simulink model "Edge_detector"  (Simulink 6.3)
settings: Solver=FixedStepDiscrete  SolverMode=SingleTasking  StartTime=0.0  StopTime=307201.0  RelTol=1e-3
InitFcn:
  | ed_in_script
  | %% DSPBuilder Start
  | alt_dspbuilder_update_model(bdroot)
  | %% DSPBuilder End
StopFcn:
  | ed_out_script
libraries: allblocks_alteradspbuilder2 x46
settings Model: LastModifiedBy=LKONG
settings DataIOCC: SignalLoggingName=sigsOut
settings OptimizationCC: InlineInvariantSignals=on
settings DebuggingCC: SolverPrmCheckMsg=none
settings HardwareCC: TargetUnknown=on

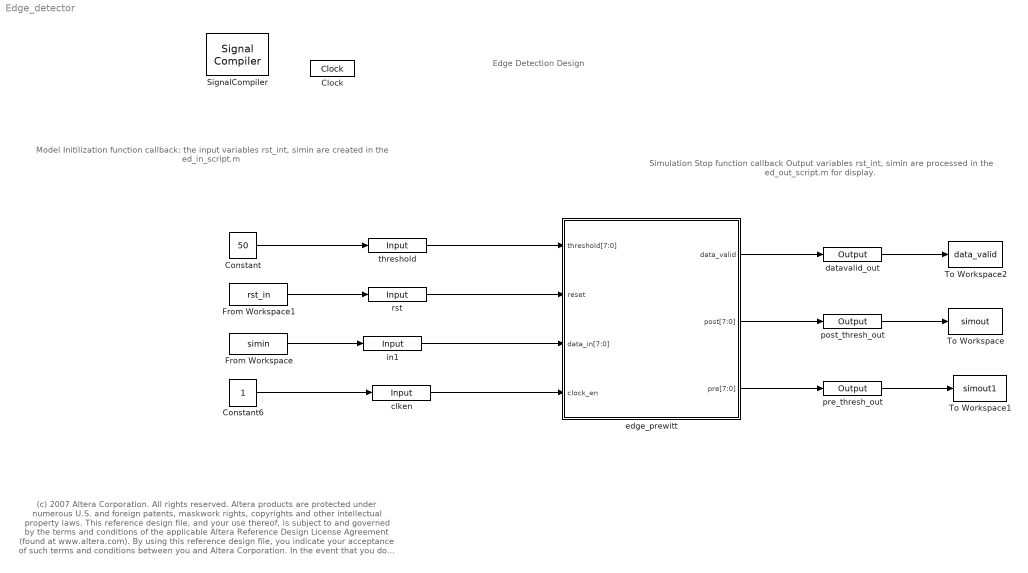
== system Edge_detector ==
  note: Edge Detection Design
  note: (c) 2007 Altera Corporation. All rights reserved.  Altera products are protected under numerous U.S. and foreign patents, maskwork rights, copyrights and other intellectual property laws.
      | This reference design file, and your use thereof, is subject to and governed by the terms and conditions of the applicable Altera Reference Design License Agreement (found at www.altera.com).
      | By using this reference design file, you indicate your acceptance of such terms and conditions between you and Altera Corporation.
      | In the event that you do not agree with such terms and conditions, you may not use the reference design file and please promptly destroy any copies you have made.
      | This reference design file being provided on an "as-is" basis and as an accommodation and therefore all warranties, representations or guarantees of any kind (whether express, implied or statutory)
      | including, without limitation, warranties of merchantability, non-infringement, or fitness for a particular purpose, are specifically disclaimed.
      | By making this reference design file available, Altera expressly does not recommend, suggest or require that this reference design file be used in combination with any other product not provided by Altera
  note: Model Initilization function callback:
      | the input  variables rst_int, simin
      | are created in the ed_in_script.m
  note: Simulation Stop function callback
      | Output  variables rst_int, simin
      | are processed in the ed_out_script.m
      | for display.
  Clock : allblocks_alteradspbuilder2/Clock  ClockPeriod=100  ClockPeriodUnit=ns  SampleTime=1  SimulationStartCycle=5  PhaseOffset=0  Reset=aclr  ResetType=Active Low  Export=off
  Constant : Constant  Value=50
  Constant6 : Constant
  From Workspace : FromWorkspace  VariableName=simin  SampleTime=1
  From Workspace1 : FromWorkspace  VariableName=rst_in  SampleTime=1
  SignalCompiler : allblocks_alteradspbuilder2/Signal Compiler  DeviceFamily=Stratix III  DeviceName=AUTO  EnableSignalTap=off  SignalTapDepth=1024  UseBoardBlock=off  StpUseDefaultClock=on  StpClock=clock
  To Workspace : ToWorkspace  VariableName=simout  SaveFormat=Array
  To Workspace1 : ToWorkspace  VariableName=simout1  SaveFormat=Array
  To Workspace2 : ToWorkspace  VariableName=data_valid  SaveFormat=Array
  clken : allblocks_alteradspbuilder2/Input  iofile=d:\wsTrunk\workspace\Documentation\DesignExamples\Demos\Video\EdgeDetection\tb_Edge_detector\Edge_detector_clken.salt  BusType=Single Bit  bwl=1  bwr=0  SpecifyClock=off  PORTTYPE=Input
  datavalid_out : allblocks_alteradspbuilder2/Output  iofile=d:\wsTrunk\workspace\Documentation\DesignExamples\Demos\Video\EdgeDetection\tb_Edge_detector\Edge_detector_datavalid_out.capture  BusType=Single Bit  bwl=1  bwr=0  PORTTYPE=Output
  edge_prewitt : Subsystem
      mask Type: SubSystem AlteraBlockSet
  in1 : allblocks_alteradspbuilder2/Input  iofile=d:\wsTrunk\workspace\Documentation\DesignExamples\Demos\Video\EdgeDetection\tb_Edge_detector\Edge_detector_in1.salt  BusType=Unsigned Integer  bwl=8  bwr=0  SpecifyClock=off  PORTTYPE=Input
  post_thresh_out : allblocks_alteradspbuilder2/Output  iofile=d:\wsTrunk\workspace\Documentation\DesignExamples\Demos\Video\EdgeDetection\tb_Edge_detector\Edge_detector_post_thresh_out.capture  BusType=Unsigned Integer  bwl=8  bwr=0  PORTTYPE=Output
  pre_thresh_out : allblocks_alteradspbuilder2/Output  iofile=d:\wsTrunk\workspace\Documentation\DesignExamples\Demos\Video\EdgeDetection\tb_Edge_detector\Edge_detector_pre_thresh_out.capture  BusType=Unsigned Integer  bwl=8  bwr=0  PORTTYPE=Output
  rst : allblocks_alteradspbuilder2/Input  iofile=d:\wsTrunk\workspace\Documentation\DesignExamples\Demos\Video\EdgeDetection\tb_Edge_detector\Edge_detector_rst.salt  BusType=Single Bit  bwl=1  bwr=0  SpecifyClock=off  PORTTYPE=Input
  threshold : allblocks_alteradspbuilder2/Input  iofile=d:\wsTrunk\workspace\Documentation\DesignExamples\Demos\Video\EdgeDetection\tb_Edge_detector\Edge_detector_threshold.salt  BusType=Unsigned Integer  bwl=8  bwr=0  SpecifyClock=off  PORTTYPE=Input
  wires:
  Constant6/1 -> clken/1
  Constant/1 -> threshold/1
  From Workspace1/1 -> rst/1
  clken/1 -> edge_prewitt/4(clock_en)
  From Workspace/1 -> in1/1
  in1/1 -> edge_prewitt/3(data_in[7:0])
  rst/1 -> edge_prewitt/2(reset)
  threshold/1 -> edge_prewitt/1(threshold[7:0])
  datavalid_out/1 -> To Workspace2/1
  edge_prewitt/2(post[7:0]) -> post_thresh_out/1
  edge_prewitt/1(data_valid) -> datavalid_out/1
  pre_thresh_out/1 -> To Workspace1/1
  post_thresh_out/1 -> To Workspace/1
  edge_prewitt/3(pre[7:0]) -> pre_thresh_out/1

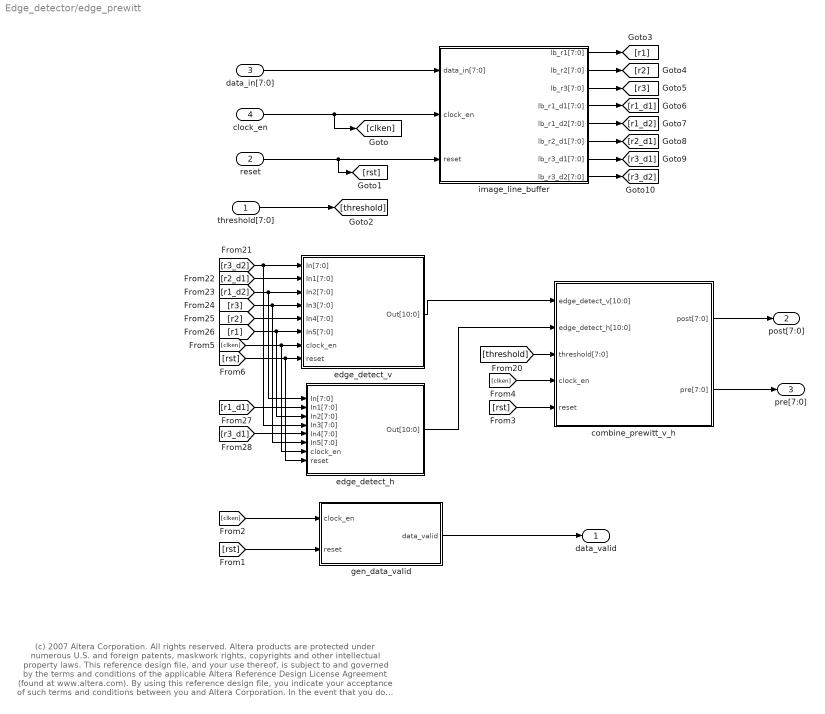
== system Edge_detector/edge_prewitt ==
  note: (c) 2007 Altera Corporation. All rights reserved.  Altera products are protected under numerous U.S. and foreign patents, maskwork rights, copyrights and other intellectual property laws.
      | This reference design file, and your use thereof, is subject to and governed by the terms and conditions of the applicable Altera Reference Design License Agreement (found at www.altera.com).
      | By using this reference design file, you indicate your acceptance of such terms and conditions between you and Altera Corporation.
      | In the event that you do not agree with such terms and conditions, you may not use the reference design file and please promptly destroy any copies you have made.
      | This reference design file being provided on an "as-is" basis and as an accommodation and therefore all warranties, representations or guarantees of any kind (whether express, implied or statutory)
      | including, without limitation, warranties of merchantability, non-infringement, or fitness for a particular purpose, are specifically disclaimed.
      | By making this reference design file available, Altera expressly does not recommend, suggest or require that this reference design file be used in combination with any other product not provided by Altera
  threshold[7:0] : Inport
  reset : Inport  Port=2
  data_in[7:0] : Inport  Port=3
  clock_en : Inport  Port=4
  combine_prewitt_v_h : Subsystem
      mask Type: SubSystem AlteraBlockSet
  edge_detect_h : Subsystem  AncestorBlock=ALTELINK/AltLab/HDL SubSystem
      mask Type: SubSystem AlteraBlockSet
  edge_detect_v : Subsystem  AncestorBlock=ALTELINK/AltLab/HDL SubSystem
      mask Type: SubSystem AlteraBlockSet
  gen_data_valid : Subsystem
      mask Type: SubSystem AlteraBlockSet
  image_line_buffer : Subsystem
      mask Type: SubSystem AlteraBlockSet
  data_valid : Outport
  post[7:0] : Outport  Port=2
  pre[7:0] : Outport  Port=3
  wires:
  threshold[7:0]/1 -> [threshold]
  edge_detect_v/1(Out[10:0]) -> combine_prewitt_v_h/1(edge_detect_v[10:0])
  edge_detect_h/1(Out[10:0]) -> combine_prewitt_v_h/2(edge_detect_h[10:0])
  [r3_d2] -> edge_detect_v/1(In[7:0]), edge_detect_h/4(In3[7:0])
  [r2_d1] -> edge_detect_v/2(In1[7:0])
  [r1_d2] -> edge_detect_v/3(In2[7:0]), edge_detect_h/1(In[7:0])
  [r3] -> edge_detect_v/4(In3[7:0]), edge_detect_h/6(In5[7:0])
  [r2] -> edge_detect_v/5(In4[7:0])
  [r1] -> edge_detect_v/6(In5[7:0]), edge_detect_h/3(In2[7:0])
  [r1_d1] -> edge_detect_h/2(In1[7:0])
  [r3_d1] -> edge_detect_h/5(In4[7:0])
  gen_data_valid/1(data_valid) -> data_valid/1
  image_line_buffer/1(lb_r1[7:0]) -> [r1]
  image_line_buffer/2(lb_r2[7:0]) -> [r2]
  image_line_buffer/3(lb_r3[7:0]) -> [r3]
  image_line_buffer/4(lb_r1_d1[7:0]) -> [r1_d1]
  image_line_buffer/5(lb_r1_d2[7:0]) -> [r1_d2]
  image_line_buffer/6(lb_r2_d1[7:0]) -> [r2_d1]
  image_line_buffer/7(lb_r3_d1[7:0]) -> [r3_d1]
  image_line_buffer/8(lb_r3_d2[7:0]) -> [r3_d2]
  [clken] -> gen_data_valid/1(clock_en)
  [rst] -> gen_data_valid/2(reset)
  [threshold] -> combine_prewitt_v_h/3(threshold[7:0])
  [clken] -> combine_prewitt_v_h/4(clock_en)
  [rst] -> combine_prewitt_v_h/5(reset)
  combine_prewitt_v_h/2(pre[7:0]) -> pre[7:0]/1
  combine_prewitt_v_h/1(post[7:0]) -> post[7:0]/1
  reset/1 -> image_line_buffer/3(reset), [rst]
  data_in[7:0]/1 -> image_line_buffer/1(data_in[7:0])
  clock_en/1 -> image_line_buffer/2(clock_en), [clken]
  [clken] -> edge_detect_v/7(clock_en), edge_detect_h/7(clock_en)
  [rst] -> edge_detect_v/8(reset), edge_detect_h/8(reset)

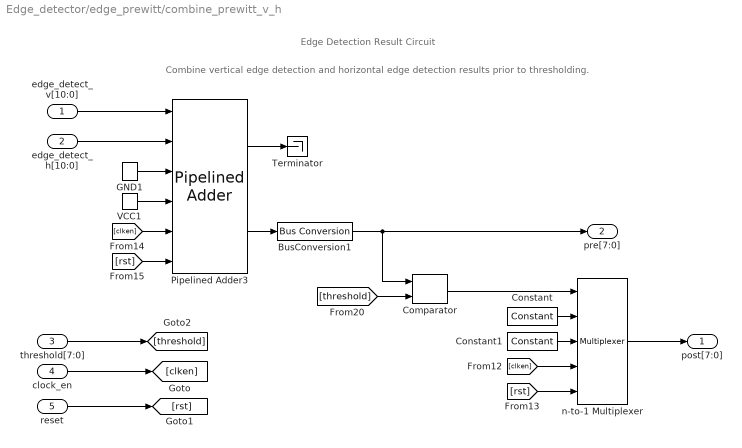
== system Edge_detector/edge_prewitt/combine_prewitt_v_h ==
  note: Combine vertical edge detection and horizontal edge detection results prior to thresholding.
  note: Edge Detection Result Circuit
  edge_detect_v[10:0] : Inport
  edge_detect_h[10:0] : Inport  Port=2
  threshold[7:0] : Inport  Port=3
  clock_en : Inport  Port=4
  reset : Inport  Port=5
  BusConversion1 : allblocks_alteradspbuilder2/Bus Conversion  BusType=Unsigned Integer  ibwl=11  ibwr=0  bwl=8  bwr=0  bitToConnectToOutputLSB=0  round=off  saturate=on
  Comparator : allblocks_alteradspbuilder2/Comparator  direction=a < b
  Constant : allblocks_alteradspbuilder2/Constant  mask_cst=255  BusType=Unsigned Integer  bwl=8  bwr=0  SpecifyClock=off
  Constant1 : allblocks_alteradspbuilder2/Constant  mask_cst=0  BusType=Unsigned Integer  bwl=8  bwr=0  SpecifyClock=off
  GND1 : allblocks_alteradspbuilder2/GND  SpecifyClock=off
  Pipelined Adder3 : allblocks_alteradspbuilder2/Pipelined Adder  BusType=Unsigned Integer  bwl=11  bwr=0  pipeline=1  AddSubDirection=ADD  use_cin=on  use_ovl=on  use_addsub=on  use_ena=on  use_aclr=on
  Terminator : Terminator
  VCC1 : allblocks_alteradspbuilder2/VCC  SpecifyClock=off
  n-to-1 Multiplexer : allblocks_alteradspbuilder2/Multiplexer  numInputs=2  pipeline=1  oneHot=off  use_ena=on  use_aclr=on
  post[7:0] : Outport
  pre[7:0] : Outport  Port=2
  wires:
  Comparator/1 -> n-to-1 Multiplexer/1
  Constant/1 -> n-to-1 Multiplexer/2
  Constant1/1 -> n-to-1 Multiplexer/3
  BusConversion1/1 -> Comparator/1, pre[7:0]/1
  [clken] -> n-to-1 Multiplexer/4
  [rst] -> n-to-1 Multiplexer/5
  Pipelined Adder3/2 -> BusConversion1/1
  GND1/1 -> Pipelined Adder3/3
  VCC1/1 -> Pipelined Adder3/4
  [clken] -> Pipelined Adder3/5
  [rst] -> Pipelined Adder3/6
  edge_detect_h[10:0]/1 -> Pipelined Adder3/2
  threshold[7:0]/1 -> [threshold]
  reset/1 -> [rst]
  n-to-1 Multiplexer/1 -> post[7:0]/1
  clock_en/1 -> [clken]
  [threshold] -> Comparator/2
  Pipelined Adder3/1 -> Terminator/1
  edge_detect_v[10:0]/1 -> Pipelined Adder3/1

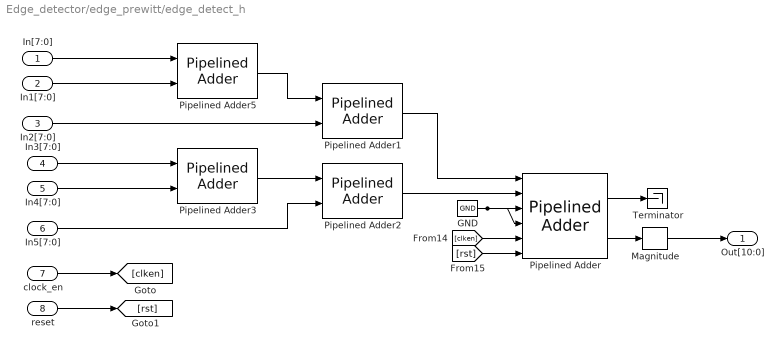
== system Edge_detector/edge_prewitt/edge_detect_h ==
  In[7:0] : Inport
  In1[7:0] : Inport  Port=2
  In2[7:0] : Inport  Port=3
  In3[7:0] : Inport  Port=4
  In4[7:0] : Inport  Port=5
  In5[7:0] : Inport  Port=6
  clock_en : Inport  Port=7
  reset : Inport  Port=8
  GND : allblocks_alteradspbuilder2/GND  SpecifyClock=off
  Magnitude : allblocks_alteradspbuilder2/Magnitude
  Pipelined Adder : allblocks_alteradspbuilder2/Pipelined Adder  BusType=Signed Integer  bwl=11  bwr=0  pipeline=1  AddSubDirection=ADD  use_cin=on  use_ovl=on  use_addsub=on  use_ena=on  use_aclr=on
  Pipelined Adder1 : allblocks_alteradspbuilder2/Pipelined Adder  BusType=Unsigned Integer  bwl=10  bwr=0  pipeline=0  AddSubDirection=ADD  use_cin=off  use_ovl=off  use_addsub=off  use_ena=off  use_aclr=off
  Pipelined Adder2 : allblocks_alteradspbuilder2/Pipelined Adder  BusType=Unsigned Integer  bwl=10  bwr=0  pipeline=0  AddSubDirection=ADD  use_cin=off  use_ovl=off  use_addsub=off  use_ena=off  use_aclr=off
  Pipelined Adder3 : allblocks_alteradspbuilder2/Pipelined Adder  BusType=Unsigned Integer  bwl=9  bwr=0  pipeline=0  AddSubDirection=ADD  use_cin=off  use_ovl=off  use_addsub=off  use_ena=off  use_aclr=off
  Pipelined Adder5 : allblocks_alteradspbuilder2/Pipelined Adder  BusType=Unsigned Integer  bwl=9  bwr=0  pipeline=0  AddSubDirection=ADD  use_cin=off  use_ovl=off  use_addsub=off  use_ena=off  use_aclr=off
  Terminator : Terminator
  Out[10:0] : Outport
  wires:
  In[7:0]/1 -> Pipelined Adder5/1
  In1[7:0]/1 -> Pipelined Adder5/2
  In2[7:0]/1 -> Pipelined Adder1/2
  Pipelined Adder5/1 -> Pipelined Adder1/1
  In3[7:0]/1 -> Pipelined Adder3/1
  In4[7:0]/1 -> Pipelined Adder3/2
  Pipelined Adder3/1 -> Pipelined Adder2/1
  Pipelined Adder1/1 -> Pipelined Adder/1
  Pipelined Adder2/1 -> Pipelined Adder/2
  Magnitude/1 -> Out[10:0]/1
  GND/1 -> Pipelined Adder/3, Pipelined Adder/4
  In5[7:0]/1 -> Pipelined Adder2/2
  reset/1 -> [rst]
  clock_en/1 -> [clken]
  Pipelined Adder/2 -> Magnitude/1
  [clken] -> Pipelined Adder/5
  [rst] -> Pipelined Adder/6
  Pipelined Adder/1 -> Terminator/1

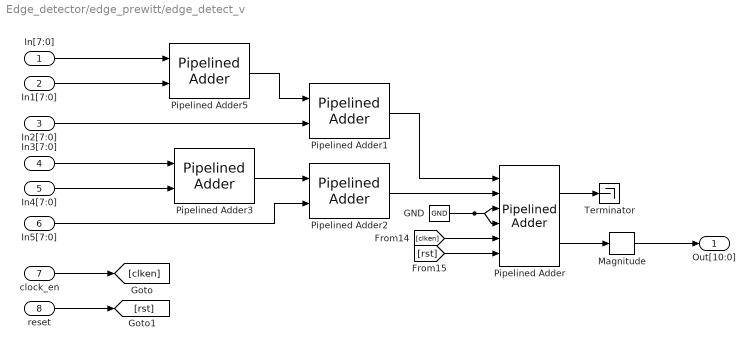
== system Edge_detector/edge_prewitt/edge_detect_v ==
  In[7:0] : Inport
  In1[7:0] : Inport  Port=2
  In2[7:0] : Inport  Port=3
  In3[7:0] : Inport  Port=4
  In4[7:0] : Inport  Port=5
  In5[7:0] : Inport  Port=6
  clock_en : Inport  Port=7
  reset : Inport  Port=8
  GND : allblocks_alteradspbuilder2/GND  SpecifyClock=off
  Magnitude : allblocks_alteradspbuilder2/Magnitude
  Pipelined Adder : allblocks_alteradspbuilder2/Pipelined Adder  BusType=Signed Integer  bwl=11  bwr=0  pipeline=1  AddSubDirection=ADD  use_cin=on  use_ovl=on  use_addsub=on  use_ena=on  use_aclr=on
  Pipelined Adder1 : allblocks_alteradspbuilder2/Pipelined Adder  BusType=Unsigned Integer  bwl=10  bwr=0  pipeline=0  AddSubDirection=ADD  use_cin=off  use_ovl=off  use_addsub=off  use_ena=off  use_aclr=off
  Pipelined Adder2 : allblocks_alteradspbuilder2/Pipelined Adder  BusType=Unsigned Integer  bwl=10  bwr=0  pipeline=0  AddSubDirection=ADD  use_cin=off  use_ovl=off  use_addsub=off  use_ena=off  use_aclr=off
  Pipelined Adder3 : allblocks_alteradspbuilder2/Pipelined Adder  BusType=Unsigned Integer  bwl=9  bwr=0  pipeline=0  AddSubDirection=ADD  use_cin=off  use_ovl=off  use_addsub=off  use_ena=off  use_aclr=off
  Pipelined Adder5 : allblocks_alteradspbuilder2/Pipelined Adder  BusType=Unsigned Integer  bwl=9  bwr=0  pipeline=0  AddSubDirection=ADD  use_cin=off  use_ovl=off  use_addsub=off  use_ena=off  use_aclr=off
  Terminator : Terminator
  Out[10:0] : Outport
  wires:
  In[7:0]/1 -> Pipelined Adder5/1
  In1[7:0]/1 -> Pipelined Adder5/2
  In2[7:0]/1 -> Pipelined Adder1/2
  Pipelined Adder5/1 -> Pipelined Adder1/1
  In3[7:0]/1 -> Pipelined Adder3/1
  In4[7:0]/1 -> Pipelined Adder3/2
  In5[7:0]/1 -> Pipelined Adder2/2
  Pipelined Adder3/1 -> Pipelined Adder2/1
  Pipelined Adder1/1 -> Pipelined Adder/1
  Pipelined Adder2/1 -> Pipelined Adder/2
  Magnitude/1 -> Out[10:0]/1
  GND/1 -> Pipelined Adder/3, Pipelined Adder/4
  Pipelined Adder/2 -> Magnitude/1
  reset/1 -> [rst]
  clock_en/1 -> [clken]
  [clken] -> Pipelined Adder/5
  [rst] -> Pipelined Adder/6
  Pipelined Adder/1 -> Terminator/1

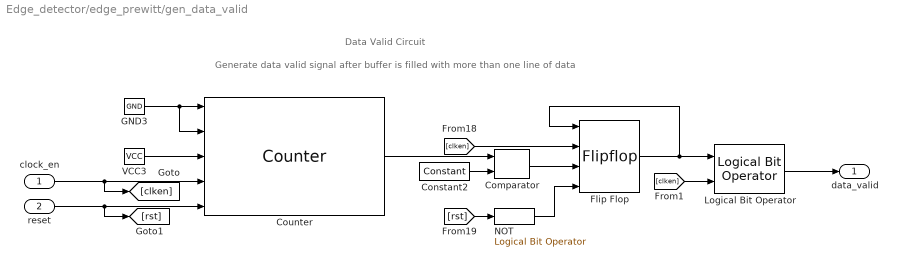
== system Edge_detector/edge_prewitt/gen_data_valid ==
  note: Generate data valid signal after buffer is filled with more than one line of data
  note: Data Valid Circuit
  clock_en : Inport
  reset : Inport  Port=2
  Comparator : allblocks_alteradspbuilder2/Comparator  direction=a < b
  Constant2 : allblocks_alteradspbuilder2/Constant  mask_cst=640+3  BusType=Unsigned Integer  bwl=12  bwr=0  SpecifyClock=off
  Counter : allblocks_alteradspbuilder2/Counter  BusType=Unsigned Integer  bwl=13  bwr=0  use_modulo=on  modulo=8*640  SpecifyClock=off  direction=Use Direction Port (updown)  use_sload=on  use_sset=off  svalue=1  use_clk_ena=off  use_ena=on  use_sclr=on
  Flip Flop : allblocks_alteradspbuilder2/Flipflop  mode=DFFE  BusType=Signed Fractional  bwl=1  bwr=1
  GND3 : allblocks_alteradspbuilder2/GND  SpecifyClock=off
  Logical Bit Operator : allblocks_alteradspbuilder2/Logical Bit Operator  LogicalOperator=AND  user_inputs=2
  NOT : allblocks_alteradspbuilder2/Logical Bit Operator  LogicalOperator=NOT  user_inputs=2
  VCC3 : allblocks_alteradspbuilder2/VCC  SpecifyClock=off
  data_valid : Outport
  wires:
  Counter/1 -> Comparator/1
  Comparator/1 -> Flip Flop/3
  [clken] -> Flip Flop/2
  NOT/1 -> Flip Flop/4
  [rst] -> NOT/1
  Flip Flop/1 -> Flip Flop/1, Logical Bit Operator/1
  Constant2/1 -> Comparator/2
  VCC3/1 -> Counter/3
  clock_en/1 -> Counter/4, [clken]
  reset/1 -> Counter/5, [rst]
  Logical Bit Operator/1 -> data_valid/1
  [clken] -> Logical Bit Operator/2
  GND3/1 -> Counter/1, Counter/2

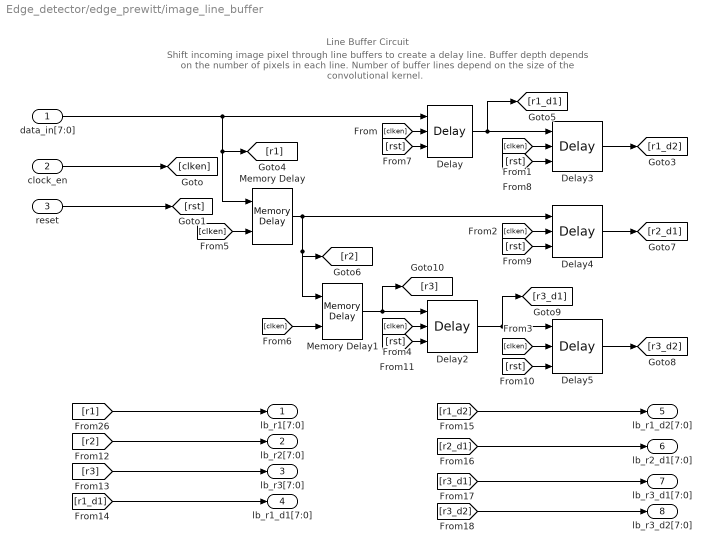
== system Edge_detector/edge_prewitt/image_line_buffer ==
  note: Shift incoming image pixel through line buffers to create a delay line.  Buffer depth depends on the number of pixels
      | in each line.  Number of buffer lines depend on the size of the convolutional kernel.
  note: Line Buffer Circuit
  data_in[7:0] : Inport
  clock_en : Inport  Port=2
  reset : Inport  Port=3
  Delay{,2..3,5} (4 alike) : allblocks_alteradspbuilder2/Delay  pipeline=1  ClockPhase=1  use_ena=on  use_sclr=on  use_init=off  reset_value=1
  Delay4 : allblocks_alteradspbuilder2/Delay  pipeline=2  ClockPhase=1  use_ena=on  use_sclr=on  use_init=off  reset_value=1
  Memory Delay : allblocks_alteradspbuilder2/Memory Delay  BusType=Inferred  bwl=8  bwr=0  pipeline=640  ram_type=AUTO  use_ena=on  use_sclr=off
  Memory Delay1 : allblocks_alteradspbuilder2/Memory Delay  BusType=Inferred  bwl=8  bwr=0  pipeline=640  ram_type=AUTO  use_ena=on  use_sclr=off
  lb_r1[7:0] : Outport
  lb_r2[7:0] : Outport  Port=2
  lb_r3[7:0] : Outport  Port=3
  lb_r1_d1[7:0] : Outport  Port=4
  lb_r1_d2[7:0] : Outport  Port=5
  lb_r2_d1[7:0] : Outport  Port=6
  lb_r3_d1[7:0] : Outport  Port=7
  lb_r3_d2[7:0] : Outport  Port=8
  wires:
  Memory Delay/1 -> Delay4/1, Memory Delay1/1, [r2]
  Memory Delay1/1 -> Delay2/1, [r3]
  [clken] -> Delay/2
  [clken] -> Delay3/2
  [clken] -> Delay4/2
  [clken] -> Delay5/2
  [clken] -> Delay2/2
  [clken] -> Memory Delay/2
  [clken] -> Memory Delay1/2
  [rst] -> Delay/3
  [rst] -> Delay3/3
  [rst] -> Delay2/3
  [rst] -> Delay4/3
  [rst] -> Delay5/3
  Delay/1 -> Delay3/1, [r1_d1]
  Delay2/1 -> Delay5/1, [r3_d1]
  data_in[7:0]/1 -> [r1], Memory Delay/1, Delay/1
  Delay3/1 -> [r1_d2]
  Delay4/1 -> [r2_d1]
  Delay5/1 -> [r3_d2]
  clock_en/1 -> [clken]
  reset/1 -> [rst]
  [r1] -> lb_r1[7:0]/1
  [r2] -> lb_r2[7:0]/1
  [r3] -> lb_r3[7:0]/1
  [r1_d1] -> lb_r1_d1[7:0]/1
  [r1_d2] -> lb_r1_d2[7:0]/1
  [r2_d1] -> lb_r2_d1[7:0]/1
  [r3_d1] -> lb_r3_d1[7:0]/1
  [r3_d2] -> lb_r3_d2[7:0]/1
